simulink model "bpsk_13_frequency"  (R2018a)
settings: Solver=VariableStepAuto  StartTime=0.0  StopTime=8  RelTol=1e-3
libraries: commrandsrc3 x1, dsparch4 x1
settings Model: Creator=hp  LastModifiedBy=hp

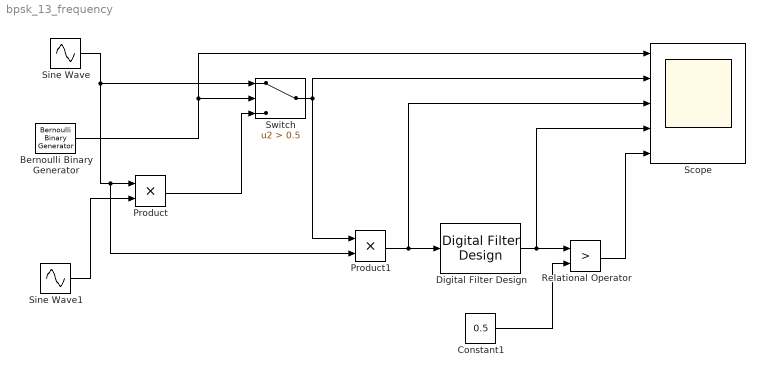
== system bpsk_13_frequency ==
  Bernoulli Binary Generator : commrandsrc3/Bernoulli Binary Generator  ProbabilityOfZero=0.5  SeedSource=Auto  Seed=0  SampleTime=1  SamplesPerFrame=1  OutputDataType=double  SimulateUsing=Interpreted execution
  Constant1 : Constant  Value=0.5
  Digital Filter Design : dsparch4/Digital Filter Design  mwdsp_browser_bugfix_var=off
  Product : Product
  Product1 : Product
  Relational Operator : RelationalOperator  Operator=>  OutDataTypeStr=boolean  RndMeth=Simplest
  Scope : Scope  NumInputPorts=5
  Sine Wave : Sin  Amplitude=2  Frequency=2*pi*13  SampleTime=0.01
  Sine Wave1 : Sin  Amplitude=2  Frequency=2*pi*13  Phase=180  SampleTime=0.01
  Switch : Switch  Criteria=u2 > Threshold  Threshold=0.5
  wires:
  Bernoulli Binary Generator/1 -> Scope/1, Switch/2
  Product/1 -> Switch/3
  Sine Wave/1 -> Product1/2, Product/1, Switch/1
  Constant1/1 -> Relational Operator/2
  Switch/1 -> Product1/1, Scope/2
  Product1/1 -> Scope/3, Digital Filter Design/1
  Relational Operator/1 -> Scope/5
  Digital Filter Design/1 -> Scope/4, Relational Operator/1
  Sine Wave1/1 -> Product/2
